simulink model "lab_2_2"  (R2024a)
settings: Solver=VariableStepAuto  StartTime=0.0  StopTime=20  MaxStep=1/128  RelTol=1e-3
settings Model: Creator=lw53894  LastModifiedBy=lw53894

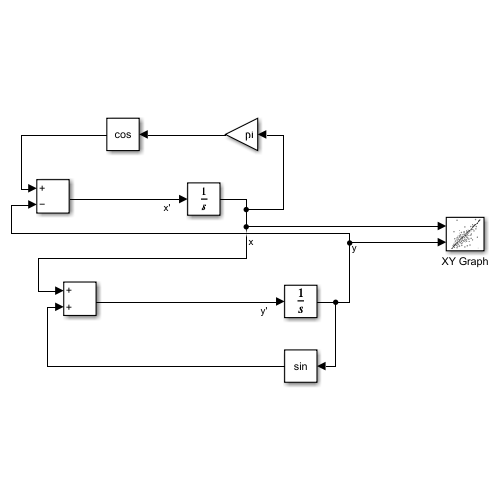
[thumbnail: Simulink's stored preview of the top-level diagram]
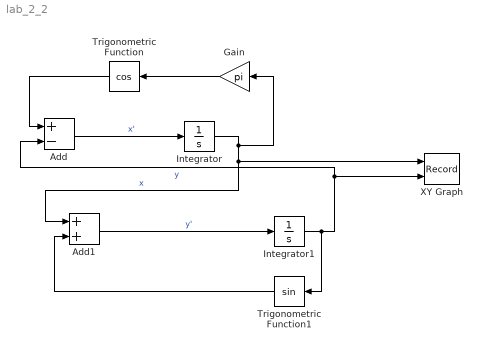
== system lab_2_2 ==
  Add : Sum  Inputs=+-
  Add1 : Sum
  Gain : Gain  Gain=pi
  Integrator : Integrator  InitialCondition=70
  Integrator1 : Integrator  InitialCondition=1
  Trigonometric Function : Trigonometry  Operator=cos
  Trigonometric Function1 : Trigonometry
  XY Graph : Record  FileSettingsInternal="{\"entries\":[{\"content\":{\"excelSettings\":{\"content\":{},\"type\":\"Streamout.ExcelSettings\"}},\"type\":\"Streamout.FileSettingStorage\",\"uuid\":\"\"}],\"packageUris\":[\"http:\\/\\/schema.mathworks.com\\/mf0\\/streamout_blocks\\/R2020a\"],\"version\":\"1.0\"}"  Layout=[1 1]  SignalsInternal="{\"entries\":[{\"content\":{\"signals\":[{\"content\":{\"blockPath\":[],\"dimensions\":[1],\"domain\":\"\",\"lineColor\":\"#a2142f\",\"plots\":[ 1 ],\"port\":1,\"sid\":[\"\"],\"signalID\":1,\"signalName\":\"x\"},\"type\":\"RecordBlkView.Signal\",\"uuid\":\"\"},{\"content\":{\"blockPath\":[],\"dimensions\":[1],\"domain\":\"\",\"lineColor\":\"#139fff\",\"plots\":[ 1 ],\"port\":2,\"sid\":[\"\"],\"signalID\":2,\"signalName\":\"y\"},\"type\":\"RecordBlkView.Signal\",\"uuid\":\"\"}]},\"type\":\"RecordBlkView.InputSignals\",\"uuid\":\"\"}],\"packageUris\":[\"http:\\/\\/schema.mathworks.com\\/mf0\\/streamout_blocks\\/R2020a\"],\"version\":\"1.0\"}"  VisualizationBindings="{\"xyplotplugin\":{\"info\":[{\"series\":[{\"bindingParametersList\":[{\"parameter\":\"X-Axis\",\"signalID\":1,\"signalName\":\"x\"},{\"parameter\":\"Y-Axis\",\"signalID\":2,\"signalName\":\"y\"}],\"seriesID\":0}],\"subplotID\":1}]}}"  CompatibilityTag=XY
  wires:
  Integrator/1 -> Gain/1, XY Graph/1, Add1/1  "x"
  Integrator1/1 -> Trigonometric Function1/1, XY Graph/2, Add/2  "y"
  Add/1 -> Integrator/1  "x'"
  Add1/1 -> Integrator1/1  "y'"
  Gain/1 -> Trigonometric Function/1
  Trigonometric Function/1 -> Add/1
  Trigonometric Function1/1 -> Add1/2
